simulink model "JT60_RCB_ACB-"  (R2015a)
settings: Solver=ode15s  StartTime=0.0  StopTime=1e3  MaxStep=1e2  RelTol=1e-3
libraries: simCryogenics_lib x146, nesl_utility x101
settings Model: Creator=GM246266  LastModifiedBy=FB229602
settings SimscapeCC: SimscapeLogType=all

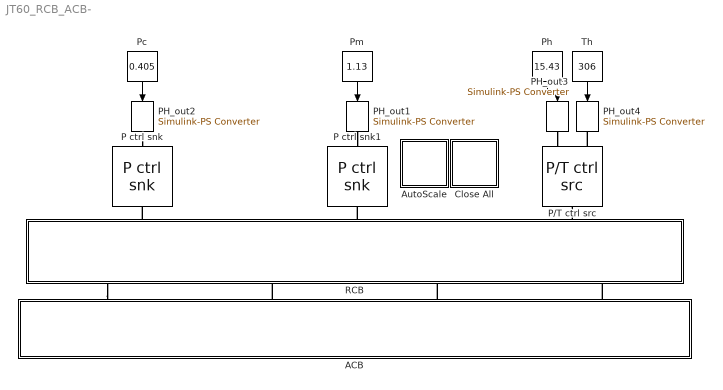
== system JT60_RCB_ACB- ==
  ACB : Subsystem
  AutoScale : Subsystem
      settings: OpenFcn=|
      | set(0, 'showhiddenhandles', 'on')
      | 
      | scope = findobj(0, 'Tag', 'SIMULINK_SIMSCOPE_FIGURE');
      | 
      | for i=1:length(scope)
      |   simscope('ScopeBar', 'ActionIcon', 'Find',     scope(i))
      | end
      | 
      | set(0, 'showhiddenhandles', 'off')
      mask Display: disp('Auto\nScale\nScope')
  Close All : Subsystem
      settings: OpenFcn=|
      | set(0, 'showhiddenhandles', 'on')
      | scope = findobj(0, 'Tag','SIMULINK_SIMSCOPE_FIGURE');
      | close(scope)
      | set(0, 'showhiddenhandles', 'off')
      mask Display: disp('Close\nAll\nScope')
  P ctrl snk : simCryogenics_lib/Sources_Sinks/P ctrl snk
  P ctrl snk1 : simCryogenics_lib/Sources_Sinks/P ctrl snk
  P/T ctrl src : simCryogenics_lib/Sources_Sinks/P//T ctrl src
  PH_out1 : nesl_utility/Simulink-PS Converter  PhysicalDomain=network_engine_domain  SubClassName=ps_input  LeftPortType=input  RightPortType=output  PseudoPeriodic=off  Frequencies=[]  NoiseDistribution=none  NoiseParameters=[]  Unit=bar  AffineConversion=off  InputFiltering=off  SimscapeFilterOrder=1  InputFilterTimeConstant=0.001  UdotUserProvided=1
  PH_out2 : nesl_utility/Simulink-PS Converter  PhysicalDomain=network_engine_domain  SubClassName=ps_input  LeftPortType=input  RightPortType=output  PseudoPeriodic=off  Frequencies=[]  NoiseDistribution=none  NoiseParameters=[]  Unit=bar  AffineConversion=off  InputFiltering=off  SimscapeFilterOrder=1  InputFilterTimeConstant=0.001  UdotUserProvided=1
  PH_out3 : nesl_utility/Simulink-PS Converter  PhysicalDomain=network_engine_domain  SubClassName=ps_input  LeftPortType=input  RightPortType=output  PseudoPeriodic=off  Frequencies=[]  NoiseDistribution=none  NoiseParameters=[]  Unit=bar  AffineConversion=off  InputFiltering=off  SimscapeFilterOrder=1  InputFilterTimeConstant=0.001  UdotUserProvided=1
  PH_out4 : nesl_utility/Simulink-PS Converter  PhysicalDomain=network_engine_domain  SubClassName=ps_input  LeftPortType=input  RightPortType=output  PseudoPeriodic=off  Frequencies=[]  NoiseDistribution=none  NoiseParameters=[]  Unit=K  AffineConversion=off  InputFiltering=off  SimscapeFilterOrder=1  InputFilterTimeConstant=0.001  UdotUserProvided=1
  Pc : Constant  Value=0.405
  Ph : Constant  Value=15.43
  Pm : Constant  Value=1.13
  RCB : Subsystem
  Th : Constant  Value=306
  wires:
  Th/1 -> PH_out4/1
  Ph/1 -> PH_out3/1
  Pm/1 -> PH_out1/1
  Pc/1 -> PH_out2/1
  connections:
  PH_out2/RConn1 -- P ctrl snk/LConn1
  PH_out1/RConn1 -- P ctrl snk1/LConn1
  PH_out3/RConn1 -- P/T ctrl src/LConn1
  P/T ctrl src/LConn2 -- PH_out4/RConn1
  RCB/RConn2 -- P ctrl snk1/RConn1
  RCB/RConn3 -- P/T ctrl src/RConn1
  RCB/RConn1 -- P ctrl snk/RConn1
  RCB/LConn1 -- ACB/RConn1
  ACB/RConn2 -- RCB/LConn2
  ACB/RConn3 -- RCB/LConn3
  ACB/RConn4 -- RCB/LConn4

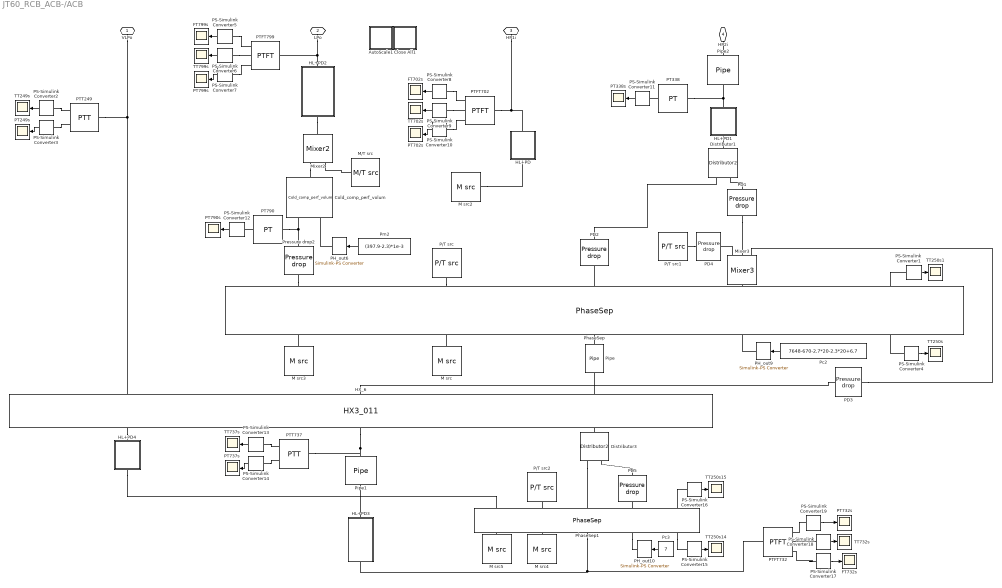
== system JT60_RCB_ACB-/ACB ==
  AutoScale1 : Subsystem
      settings: OpenFcn=|
      | set(0, 'showhiddenhandles', 'on')
      | 
      | scope = findobj(0, 'Tag', 'SIMULINK_SIMSCOPE_FIGURE');
      | 
      | for i=1:length(scope)
      |   simscope('ScopeBar', 'ActionIcon', 'Find',     scope(i))
      | end
      | 
      | set(0, 'showhiddenhandles', 'off')
      mask Display: disp('Auto\nScale\nScope')
  Close All1 : Subsystem
      settings: OpenFcn=|
      | set(0, 'showhiddenhandles', 'on')
      | scope = findobj(0, 'Tag','SIMULINK_SIMSCOPE_FIGURE');
      | close(scope)
      | set(0, 'showhiddenhandles', 'off')
      mask Display: disp('Close\nAll\nScope')
  Cold_comp_perf_volum : simCryogenics_lib/Elements/Cold_comp_perf_volum  P0=1.069 bar  eta=0.68  Sin_specify=off  Sin_priority=High  Sin=0 kJ/kg  HoutIs_specify=off  HoutIs_priority=High  HoutIs=0 kJ/kg
  Distributor1 : simCryogenics_lib/Elements/Distributor2
  Distributor3 : simCryogenics_lib/Elements/Distributor2
  FT702s : Scope
      settings: SaveName=FT
  FT732s : Scope
      settings: SaveName=FT732
  FT799s : Scope
      settings: SaveName=FT799
  HL+PD : Subsystem
  HL+PD1 : Subsystem
  HL+PD2 : Subsystem
  HL+PD3 : Subsystem
  HL+PD4 : Subsystem
  HX_6 : simCryogenics_lib/Elements/HX3_011  N=10  Vh=1 m^3  Vm=1 m^3  Vc=1 m^3  M=1000 kg  Kh=0.02/0.3068 s*bar/kg  Km=0.005/0.2835 s*bar/kg  Kc=0.02/0.02334 s*bar/kg  hh_m=865.4*(0.2835)/(0.2835+0.02334) J/s/K  hh_c=865.4*(0.02334)/(0.2835+0.02334) J/s/K  hm_c=1 J/s/K  Th0=4.4 K  Ph0=4.79 bar  Mh0=0.3068 kg/s  Tm0=3.7 K  Pm0=4.2 bar  Mm0=0.2835 kg/s  Tc0=3.661 K  Pc0=0.53 bar  Mc0=0.02334 kg/s  sensh=0  sensm=1  sensc=1
  M src{,3..5} (4 alike) : simCryogenics_lib/Sources_Sinks/M src  M=0 kg/s
  M src2 : simCryogenics_lib/Sources_Sinks/M src  M=0.020 kg/s
  M/T src : simCryogenics_lib/Sources_Sinks/M//T src  M=0.0023 kg/s  T=4.784 K
  Mixer2 : simCryogenics_lib/Elements/Mixer2
  Mixer3 : simCryogenics_lib/Elements/Mixer3
  P/T src : simCryogenics_lib/Sources_Sinks/P//T src  P=1 bar  T=300 K
  P/T src1 : simCryogenics_lib/Sources_Sinks/P//T src  P=4.44 bar  T=4.407 K
  P/T src2 : simCryogenics_lib/Sources_Sinks/P//T src  P=1 bar  T=300 K
  PD1 : simCryogenics_lib/Utilities/Pressure drop  K=3.771/0.09206 s*bar/kg
  PD2 : simCryogenics_lib/Utilities/Pressure drop  K=0.07/0.3068 s*bar/kg
  PD3 : simCryogenics_lib/Utilities/Pressure drop  K=3.106/0.2835 s*bar/kg
  PD4 : simCryogenics_lib/Utilities/Pressure drop  K=3.351/0.02 s*bar/kg
  PD5 : simCryogenics_lib/Utilities/Pressure drop  K=4.240/0.02334 s*bar/kg
  PH_out10 : nesl_utility/Simulink-PS Converter  PhysicalDomain=network_engine_domain  SubClassName=ps_input  LeftPortType=input  RightPortType=output  PseudoPeriodic=off  Frequencies=[]  NoiseDistribution=none  NoiseParameters=[]  Unit=1  AffineConversion=off  InputFiltering=off  SimscapeFilterOrder=1  InputFilterTimeConstant=0.001  UdotUserProvided=1
  PH_out6 : nesl_utility/Simulink-PS Converter  PhysicalDomain=network_engine_domain  SubClassName=ps_input  LeftPortType=input  RightPortType=output  PseudoPeriodic=off  Frequencies=[]  NoiseDistribution=none  NoiseParameters=[]  Unit=1  AffineConversion=off  InputFiltering=off  SimscapeFilterOrder=1  InputFilterTimeConstant=0.001  UdotUserProvided=1
  PH_out9 : nesl_utility/Simulink-PS Converter  PhysicalDomain=network_engine_domain  SubClassName=ps_input  LeftPortType=input  RightPortType=output  PseudoPeriodic=off  Frequencies=[]  NoiseDistribution=none  NoiseParameters=[]  Unit=1  AffineConversion=off  InputFiltering=off  SimscapeFilterOrder=1  InputFilterTimeConstant=0.001  UdotUserProvided=1
  PS-Simulink Converter{1..19} (19 alike) : nesl_utility/PS-Simulink Converter  PhysicalDomain=network_engine_domain  SubClassName=ps_output  LeftPortType=input  RightPortType=output  PseudoPeriodic=off  Frequencies=[]  Unit=1  AffineConversion=off
  PT249s : Scope
      settings: SaveName=PT
  PT338 : simCryogenics_lib/Sensors/PT
  PT338s : Scope
      settings: SaveName=PT1
  PT702s : Scope
      settings: SaveName=PT2
  PT732s : Scope
      settings: SaveName=PT732
  PT737s : Scope
      settings: SaveName=PT737
  PT790 : simCryogenics_lib/Sensors/PT
  PT790s : Scope
      settings: YMin=0  YMax=2.5  SaveName=PT790
  PT799s : Scope
      settings: SaveName=PT3
  PTFT702 : simCryogenics_lib/Sensors/PTFT
  PTFT732 : simCryogenics_lib/Sensors/PTFT
  PTFT799 : simCryogenics_lib/Sensors/PTFT
  PTT249 : simCryogenics_lib/Sensors/PTT
  PTT737 : simCryogenics_lib/Sensors/PTT
  Pc2 : Constant  Value=7648-670-2.7*20-2.3*20+6.7
  Pc3 : Constant  Value=7
  PhaseSep : simCryogenics_lib/Elements/PhaseSep  Ideal1=1  DeltaT1=1 K  N1=1  h1=1 W/K  Ideal2=1  DeltaT2=0.1 K  N2=1  h2=1 W/K  hmax=10 m  S=10 m^2  P0=1.089 bar  h0=50
  PhaseSep1 : simCryogenics_lib/Elements/PhaseSep  Ideal1=1  DeltaT1=1 K  N1=1  h1=1 W/K  Ideal2=1  DeltaT2=0.1 K  N2=1  h2=1 W/K  hmax=10 m  S=10 m^2  P0=0.53 bar  h0=50
  Pipe : simCryogenics_lib/Elements/Pipe  Vol=0.01 m^3  Ideal=1  P0=4.79 bar  T0=4.16 K
  Pipe1 : simCryogenics_lib/Elements/Pipe  Vol=0.01 m^3  Ideal=1  P0=4.195 bar  T0=4.16 K
  Pipe2 : simCryogenics_lib/Elements/Pipe  Vol=0.01 m^3  Ideal=1  P0=4.87 bar  T0=4.91 K
  Pm2 : Constant  Value=(397.9-2.3)*1e-3
  Pressure drop2 : simCryogenics_lib/Utilities/Pressure drop  K=0.02/((397.9-2.3)*1e-3) s*bar/kg
  TT249s : Scope
      settings: SaveName=TT249
  TT250s{,1,14..15} (4 alike) : Scope
      TT250s settings: TimeRange=100000  YMin=49.99  YMax=50.08000000000001  SaveName=TT
      TT250s1 settings: SaveName=TT1
      TT250s14 settings: TimeRange=24979.14205816138  YMin=48.2  YMax=49.7  SaveName=TT14
      TT250s15 settings: SaveName=TT15
  TT702s : Scope
      settings: SaveName=FT702
  TT732s : Scope
      settings: SaveName=TT732
  TT737s : Scope
      settings: SaveName=TT737
  TT799s : Scope
      settings: SaveName=TT799
  VLPo : PMIOPort  Port=1  Side=Right
  LPo : PMIOPort  Port=2  Side=Right
  HP1i : PMIOPort  Port=3  Side=Right
  HP2i : PMIOPort  Port=4  Side=Right
  wires:
  PS-Simulink Converter8/1 -> FT702s/1
  PS-Simulink Converter1/1 -> TT250s1/1
  Pc2/1 -> PH_out9/1
  PS-Simulink Converter4/1 -> TT250s/1
  PS-Simulink Converter15/1 -> TT250s14/1
  PS-Simulink Converter3/1 -> PT249s/1
  PS-Simulink Converter16/1 -> TT250s15/1
  PS-Simulink Converter6/1 -> TT799s/1
  PS-Simulink Converter2/1 -> TT249s/1
  Pc3/1 -> PH_out10/1
  PS-Simulink Converter5/1 -> FT799s/1
  PS-Simulink Converter9/1 -> TT702s/1
  PS-Simulink Converter13/1 -> TT737s/1
  PS-Simulink Converter12/1 -> PT790s/1
  PS-Simulink Converter11/1 -> PT338s/1
  PS-Simulink Converter7/1 -> PT799s/1
  PS-Simulink Converter18/1 -> TT732s/1
  PS-Simulink Converter14/1 -> PT737s/1
  PS-Simulink Converter19/1 -> PT732s/1
  PS-Simulink Converter10/1 -> PT702s/1
  PS-Simulink Converter17/1 -> FT732s/1
  Pm2/1 -> PH_out6/1
  connections:
  PT338/LConn1 -- HL+PD1/LConn1 -- Pipe2/RConn1
  HL+PD2/RConn1 -- LPo/RConn1 -- PTFT799/LConn1
  PTFT702/LConn1 -- HP1i/RConn1 -- HL+PD/LConn1
  PTT249/LConn1 -- HX_6/LConn1 -- VLPo/RConn1
  P/T src/RConn1 -- PhaseSep/LConn2
  HL+PD3/RConn1 -- Pipe1/LConn1
  HL+PD3/LConn1 -- PhaseSep1/RConn3 -- PTFT732/LConn1
  Mixer3/RConn1 -- PhaseSep/LConn4
  Cold_comp_perf_volum/LConn1 -- PT790/LConn1 -- Pressure drop2/RConn1
  HX_6/LConn3 -- Pipe/RConn1
  Distributor3/RConn2 -- PhaseSep1/LConn3
  PS-Simulink Converter8/LConn1 -- PTFT702/RConn3
  PS-Simulink Converter7/LConn1 -- PTFT799/RConn1
  HX_6/RConn3 -- Distributor3/LConn1
  PH_out6/RConn1 -- Cold_comp_perf_volum/LConn2
  PD5/RConn1 -- PhaseSep1/LConn4
  PS-Simulink Converter2/LConn1 -- PTT249/RConn2
  PS-Simulink Converter1/LConn1 -- PhaseSep/LConn5
  HL+PD4/LConn1 -- PhaseSep1/LConn1
  Mixer3/LConn3 -- PD4/RConn1
  M src3/RConn1 -- PhaseSep/RConn1
  HX_6/LConn2 -- PD3/LConn1
  PS-Simulink Converter16/LConn1 -- PhaseSep1/LConn5
  PD5/LConn1 -- Distributor3/RConn1
  PS-Simulink Converter5/LConn1 -- PTFT799/RConn3
  PS-Simulink Converter14/LConn1 -- PTT737/RConn1
  PS-Simulink Converter3/LConn1 -- PTT249/RConn1
  P/T src2/RConn1 -- PhaseSep1/LConn2
  PT790/RConn1 -- PS-Simulink Converter12/LConn1
  Pipe/LConn1 -- PhaseSep/RConn3
  PS-Simulink Converter4/LConn1 -- PhaseSep/RConn5
  PhaseSep/LConn3 -- PD2/RConn1
  PS-Simulink Converter6/LConn1 -- PTFT799/RConn2
  PD1/RConn1 -- Mixer3/LConn2
  HX_6/RConn1 -- HL+PD4/RConn1
  PS-Simulink Converter9/LConn1 -- PTFT702/RConn2
  PS-Simulink Converter18/LConn1 -- PTFT732/RConn2
  PH_out9/RConn1 -- PhaseSep/RConn4
  M src5/RConn1 -- PhaseSep1/RConn1
  PS-Simulink Converter10/LConn1 -- PTFT702/RConn1
  Pressure drop2/LConn1 -- PhaseSep/LConn1
  PS-Simulink Converter17/LConn1 -- PTFT732/RConn3
  M src2/RConn1 -- HL+PD/RConn1
  Distributor1/RConn2 -- PD2/LConn1
  P/T src1/RConn1 -- PD4/LConn1
  M src4/RConn1 -- PhaseSep1/RConn2
  PD3/RConn1 -- Mixer3/LConn1
  PS-Simulink Converter13/LConn1 -- PTT737/RConn2
  Distributor1/LConn1 -- HL+PD1/RConn1
  PT338/RConn1 -- PS-Simulink Converter11/LConn1
  PS-Simulink Converter19/LConn1 -- PTFT732/RConn1
  PhaseSep1/RConn4 -- PH_out10/RConn1
  Mixer2/LConn1 -- Cold_comp_perf_volum/RConn1
  PD1/LConn1 -- Distributor1/RConn1
  PhaseSep1/RConn5 -- PS-Simulink Converter15/LConn1
  Pipe1/RConn1 -- HX_6/RConn2 -- PTT737/LConn1
  M src/RConn1 -- PhaseSep/RConn2
  Pipe2/LConn1 -- HP2i/RConn1
  M/T src/RConn1 -- Mixer2/LConn2
  HL+PD2/LConn1 -- Mixer2/RConn1

== system JT60_RCB_ACB-/AutoScale ==

== system JT60_RCB_ACB-/Close All ==

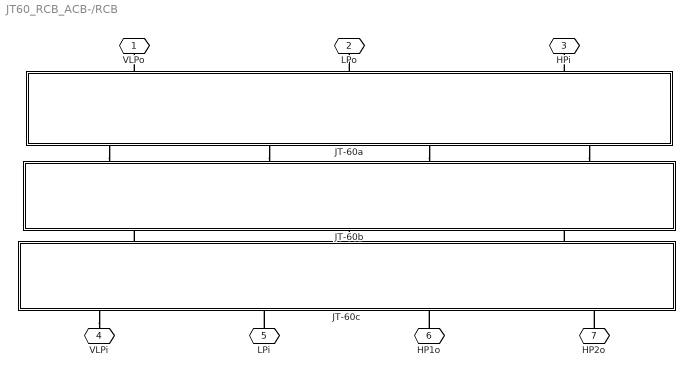
== system JT60_RCB_ACB-/RCB ==
  JT-60a : Subsystem
  JT-60b : Subsystem
  "JT-60c " : Subsystem
  VLPo : PMIOPort  Port=1  Side=Right
  LPo : PMIOPort  Port=2  Side=Right
  HPi : PMIOPort  Port=3  Side=Right
  VLPi : PMIOPort  Port=4  Side=Left
  LPi : PMIOPort  Port=5  Side=Left
  HP1o : PMIOPort  Port=6  Side=Left
  HP2o : PMIOPort  Port=7  Side=Left
  connections:
  JT-60a/LConn2 -- JT-60b/RConn2
  JT-60a/LConn3 -- JT-60b/RConn3
  JT-60a/LConn4 -- JT-60b/RConn4
  "JT-60c "/RConn2 -- JT-60b/LConn2
  "JT-60c "/RConn3 -- JT-60b/LConn3
  "JT-60c "/RConn1 -- JT-60b/LConn1
  HP2o/RConn1 -- "JT-60c "/LConn4
  "JT-60c "/LConn1 -- VLPi/RConn1
  LPi/RConn1 -- "JT-60c "/LConn2
  HP1o/RConn1 -- "JT-60c "/LConn3
  JT-60a/RConn1 -- VLPo/RConn1
  JT-60a/RConn2 -- LPo/RConn1
  JT-60a/RConn3 -- HPi/RConn1
  JT-60a/LConn1 -- JT-60b/RConn1

== system JT60_RCB_ACB-/ACB/AutoScale1 ==

== system JT60_RCB_ACB-/ACB/Close All1 ==

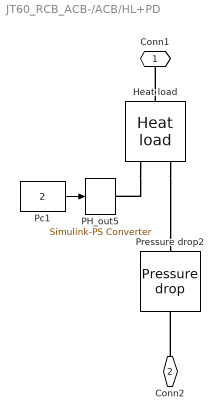
== system JT60_RCB_ACB-/ACB/HL+PD ==
  Heat load : simCryogenics_lib/Utilities/Heat load
  PH_out5 : nesl_utility/Simulink-PS Converter  PhysicalDomain=network_engine_domain  SubClassName=ps_input  LeftPortType=input  RightPortType=output  PseudoPeriodic=off  Frequencies=[]  NoiseDistribution=none  NoiseParameters=[]  Unit=J/s  AffineConversion=off  InputFiltering=off  SimscapeFilterOrder=1  InputFilterTimeConstant=0.001  UdotUserProvided=1
  Pc1 : Constant  Value=2
  Pressure drop2 : simCryogenics_lib/Utilities/Pressure drop  K=0.010/0.020 s*bar/kg
  Conn1 : PMIOPort  Port=1  Side=Right
  Conn2 : PMIOPort  Port=2  Side=Left
  wires:
  Pc1/1 -> PH_out5/1
  connections:
  Heat load/RConn1 -- Conn1/RConn1
  Conn2/RConn1 -- Pressure drop2/LConn1
  Heat load/LConn2 -- PH_out5/RConn1
  Heat load/LConn1 -- Pressure drop2/RConn1

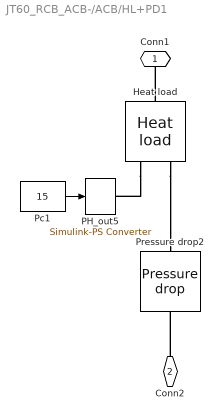
== system JT60_RCB_ACB-/ACB/HL+PD1 ==
  Heat load : simCryogenics_lib/Utilities/Heat load
  PH_out5 : nesl_utility/Simulink-PS Converter  PhysicalDomain=network_engine_domain  SubClassName=ps_input  LeftPortType=input  RightPortType=output  PseudoPeriodic=off  Frequencies=[]  NoiseDistribution=none  NoiseParameters=[]  Unit=J/s  AffineConversion=off  InputFiltering=off  SimscapeFilterOrder=1  InputFilterTimeConstant=0.001  UdotUserProvided=1
  Pc1 : Constant  Value=15
  Pressure drop2 : simCryogenics_lib/Utilities/Pressure drop  K=0.010/0.3989 s*bar/kg
  Conn1 : PMIOPort  Port=1  Side=Right
  Conn2 : PMIOPort  Port=2  Side=Left
  wires:
  Pc1/1 -> PH_out5/1
  connections:
  Heat load/RConn1 -- Conn1/RConn1
  Conn2/RConn1 -- Pressure drop2/LConn1
  Heat load/LConn2 -- PH_out5/RConn1
  Heat load/LConn1 -- Pressure drop2/RConn1

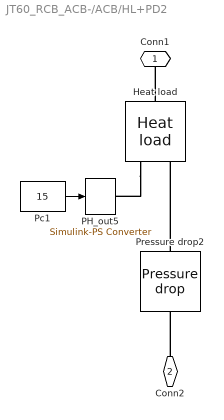
== system JT60_RCB_ACB-/ACB/HL+PD2 ==
  Heat load : simCryogenics_lib/Utilities/Heat load
  PH_out5 : nesl_utility/Simulink-PS Converter  PhysicalDomain=network_engine_domain  SubClassName=ps_input  LeftPortType=input  RightPortType=output  PseudoPeriodic=off  Frequencies=[]  NoiseDistribution=none  NoiseParameters=[]  Unit=J/s  AffineConversion=off  InputFiltering=off  SimscapeFilterOrder=1  InputFilterTimeConstant=0.001  UdotUserProvided=1
  Pc1 : Constant  Value=15
  Pressure drop2 : simCryogenics_lib/Utilities/Pressure drop  K=0.01/((397.9-2.3)*1e-3) s*bar/kg
  Conn1 : PMIOPort  Port=1  Side=Right
  Conn2 : PMIOPort  Port=2  Side=Left
  wires:
  Pc1/1 -> PH_out5/1
  connections:
  Heat load/RConn1 -- Conn1/RConn1
  Heat load/LConn2 -- PH_out5/RConn1
  Conn2/RConn1 -- Pressure drop2/LConn1
  Pressure drop2/RConn1 -- Heat load/LConn1

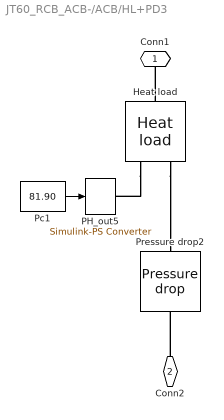
== system JT60_RCB_ACB-/ACB/HL+PD3 ==
  Heat load : simCryogenics_lib/Utilities/Heat load
  PH_out5 : nesl_utility/Simulink-PS Converter  PhysicalDomain=network_engine_domain  SubClassName=ps_input  LeftPortType=input  RightPortType=output  PseudoPeriodic=off  Frequencies=[]  NoiseDistribution=none  NoiseParameters=[]  Unit=J/s  AffineConversion=off  InputFiltering=off  SimscapeFilterOrder=1  InputFilterTimeConstant=0.001  UdotUserProvided=1
  Pc1 : Constant  Value=81.90
  Pressure drop2 : simCryogenics_lib/Utilities/Pressure drop  K=(0.5+0.07)/0.2835 s*bar/kg
  Conn1 : PMIOPort  Port=1  Side=Right
  Conn2 : PMIOPort  Port=2  Side=Left
  wires:
  Pc1/1 -> PH_out5/1
  connections:
  Heat load/LConn1 -- Pressure drop2/RConn1
  Heat load/LConn2 -- PH_out5/RConn1
  Conn2/RConn1 -- Pressure drop2/LConn1
  Heat load/RConn1 -- Conn1/RConn1

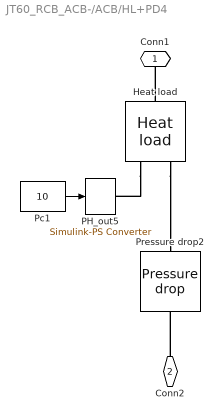
== system JT60_RCB_ACB-/ACB/HL+PD4 ==
  Heat load : simCryogenics_lib/Utilities/Heat load
  PH_out5 : nesl_utility/Simulink-PS Converter  PhysicalDomain=network_engine_domain  SubClassName=ps_input  LeftPortType=input  RightPortType=output  PseudoPeriodic=off  Frequencies=[]  NoiseDistribution=none  NoiseParameters=[]  Unit=J/s  AffineConversion=off  InputFiltering=off  SimscapeFilterOrder=1  InputFilterTimeConstant=0.001  UdotUserProvided=1
  Pc1 : Constant  Value=10
  Pressure drop2 : simCryogenics_lib/Utilities/Pressure drop  K=0.01/0.02334 s*bar/kg
  Conn1 : PMIOPort  Port=1  Side=Right
  Conn2 : PMIOPort  Port=2  Side=Left
  wires:
  Pc1/1 -> PH_out5/1
  connections:
  Heat load/LConn1 -- Pressure drop2/RConn1
  Heat load/LConn2 -- PH_out5/RConn1
  Conn2/RConn1 -- Pressure drop2/LConn1
  Heat load/RConn1 -- Conn1/RConn1

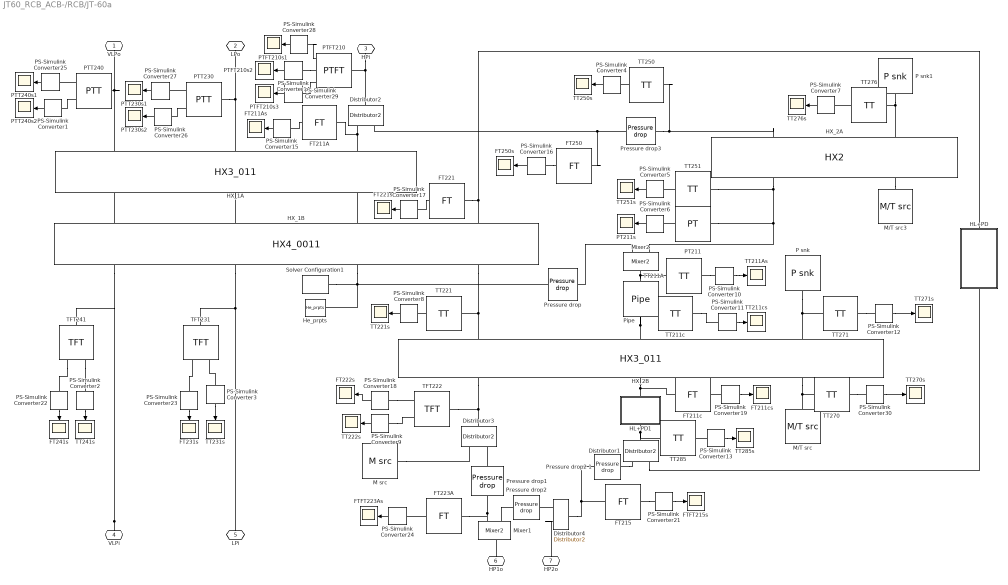
== system JT60_RCB_ACB-/RCB/JT-60a ==
  Distributor{1..4} (4 alike) : simCryogenics_lib/Elements/Distributor2
  FT211A : simCryogenics_lib/Sensors/FT
  FT211As : Scope
      settings: SaveName=FT211A
  FT211c : simCryogenics_lib/Sensors/FT
  FT211cs : Scope
      settings: SaveName=FT211c
  FT215 : simCryogenics_lib/Sensors/FT
  FT221 : simCryogenics_lib/Sensors/FT
  FT221s : Scope
      settings: SaveName=FT221
  FT222s : Scope
      settings: SaveName=FT222
  FT223A : simCryogenics_lib/Sensors/FT
  FT231s : Scope
      settings: SaveName=FT231
  FT241s : Scope
      settings: SaveName=FT241
  FT250 : simCryogenics_lib/Sensors/FT
  FT250s : Scope
      settings: SaveName=FT250
  FTFT215s : Scope
      settings: SaveName=FT215
  FTFT223As : Scope
      settings: SaveName=FT223A
  HL+PD : Subsystem
  HL+PD1 : Subsystem
  HX_1A : simCryogenics_lib/Elements/HX3_011  N=10  Vh=1 m^3  Vm=1 m^3  Vc=1 m^3  M=1000 kg  Kh=0 s*bar/kg  Km=0 s*bar/kg  Kc=0 s*bar/kg  hh_m=199100*0.585/(0.585+0.02334) J/s/K  hh_c=199100*0.02334/(0.585+0.02334) J/s/K  hm_c=1 J/s/K  Th0=306 K  Ph0=15.34 bar  Mh0=0.584 kg/s  Tm0=98 K  Pm0=1.130 bar  Mm0=0.589 kg/s  Tc0=98 K  Pc0=0.405 bar  Mc0=0.02334 kg/s  sensh=0  sensm=1  sensc=1
  HX_1B : simCryogenics_lib/Elements/HX4_0011  N=10  Vh=1 m^3  Vm=1 m^3  Vc=1 m^3  Vvc=1 m^3  M=1000 kg  Kh=0.03/0.425 s*bar/kg  Km=0.085/0.5925 s*bar/kg  Kc=0.135/0.589 s*bar/kg  Kvc=0.050/0.02334 s*bar/kg  hh_m=1 J/s/K  hh_c=17240*0.425/(0.425+0.584)*0.589/(0.589+0.02334) J/s/K  hh_vc=17240*0.425/(0.425+0.584)*0.02334/(0.589+0.02334) J/s/K  hm_c=17240*0.584/(0.425+0.584)*0.589/(0.589+0.02334) J/s/K  hm_vc=17240*0.584/(0.425+0.584)*0.02334/(0.589+0.02334) J/s/K  hc_vc=1 J/s/K  Th0=98 K  Ph0=15 bar  Mh0=0.425 kg/s  Tm0=99 K  Pm0=15 bar  Mm0=0.584 kg/s  Tc0=78 K  Pc0=1.1 bar  Mc0=0.589 kg/s  Tvc0=78 K  Pvc0=0.405 bar  Mvc0=0.02334 kg/s  sensh=0  sensm=0  sensc=1  sensvc=1
  HX_2A : simCryogenics_lib/Elements/HX2  N=10  Vh=1 m^3  Vc=1 m^3  M=1000 kg  Kh=0.05/0.04498 s*bar/kg  Kc=0 s*bar/kg  h=16470 J/s/K  Th0=300 K  Ph0=15 bar  Mc0=0.047*2 kg/s  Tc0=78 K  Pc0=1.1 bar  Mh0=0.047 kg/s
  HX_2B : simCryogenics_lib/Elements/HX3_011  N=10  Vh=1 m^3  Vm=1 m^3  Vc=1 m^3  M=1000 kg  Kh=0 s*bar/kg  Km=0.050/0.6374 s*bar/kg  Kc=0.030/0.425 s*bar/kg  hh_m=12710*0.6205/(0.6205+0.419) J/s/K  hh_c=12710*0.419/(0.6205+0.419) J/s/K  hm_c=1 J/s/K  Th0=78 K  Ph0=1.1 bar  Mh0=2 kg/s  Tm0=86.85 K  Pm0=15.33 bar  Mm0=0.6205 kg/s  Tc0=86.85 K  Pc0=15 bar  Mc0=0.419 kg/s  sensh=0  sensm=1  sensc=1
  He_prpts : simCryogenics_lib/Utilities/He_prpts  P_min=0.25 bar  T_min=3 K  T_max=320 K  P_max=20 bar  Mol=4.0026 * 10 ^ (- 3) kg/mol
  M src : simCryogenics_lib/Sources_Sinks/M src  M=6.6e-3 kg/s
  M/T src : simCryogenics_lib/Sources_Sinks/M//T src  M=4 kg/s  T=78 K
  M/T src3 : simCryogenics_lib/Sources_Sinks/M//T src  M=0.047*2 kg/s  T=78 K
  Mixer1 : simCryogenics_lib/Elements/Mixer2
  Mixer2 : simCryogenics_lib/Elements/Mixer2
  P snk : simCryogenics_lib/Sources_Sinks/P snk  P=1.1 bar
  P snk1 : simCryogenics_lib/Sources_Sinks/P snk  P=1.1 bar
  PS-Simulink Converter{1..19,21..30} (29 alike) : nesl_utility/PS-Simulink Converter  PhysicalDomain=network_engine_domain  SubClassName=ps_output  LeftPortType=input  RightPortType=output  PseudoPeriodic=off  Frequencies=[]  Unit=1  AffineConversion=off
  PT211 : simCryogenics_lib/Sensors/PT
  PT211s : Scope
      settings: SaveName=PT211
  PTFT210 : simCryogenics_lib/Sensors/PTFT
  PTFT210s1 : Scope
      settings: SaveName=FT210
  PTFT210s2 : Scope
      settings: SaveName=TT210
  PTFT210s3 : Scope
      settings: SaveName=PT210
  PTT230 : simCryogenics_lib/Sensors/PTT
  PTT230s1 : Scope
      settings: SaveName=TT230
  PTT230s2 : Scope
      settings: SaveName=PT230
  PTT240 : simCryogenics_lib/Sensors/PTT
  PTT240s1 : Scope
      settings: SaveName=TT240
  PTT240s2 : Scope
      settings: SaveName=PT240
  Pipe : simCryogenics_lib/Elements/Pipe  Vol=1 m^3  Ideal=0  P0=15.28 bar  T0=86.85 K
  Pressure drop : simCryogenics_lib/Utilities/Pressure drop  K=0.065/0.5925 s*bar/kg
  Pressure drop1 : simCryogenics_lib/Utilities/Pressure drop  K=0.010/0.4184 s*bar/kg
  "Pressure drop2 " : simCryogenics_lib/Utilities/Pressure drop  K=1.540/0.02108 s*bar/kg
  Pressure drop2 1 : simCryogenics_lib/Utilities/Pressure drop  K=0.04/0.2124 s*bar/kg
  Pressure drop3 : simCryogenics_lib/Utilities/Pressure drop  K=0.1/0.04498 s*bar/kg
  Solver Configuration1 : nesl_utility/Solver Configuration  PhysicalDomain=network_engine_domain  SubClassName=solver  LeftPortType=input  RightPortType=generic  Accelerate=off  Tones=[]  Harmonics=[]  SimulateNoise=off  Profile=off  UseLocalSampling=off  EnableSwitchedLinearOptims=on  FrequencyDomain=off  UseCCode=off  RelTol=0.001  AbsTol=1e-06  MinStep=1e-09  ToWorkspace=off  RevertToSquareIcSolve=off  NumHomotopyIterations=100  DoDC=off  ResidualTolerance=1e-09  UseLocalSolver=off  LocalSolverChoice=NE_BACKWARD_EULER_ADVANCER  LocalSolverSampleTime=5  DoFixedCost=off  MaxNonlinIter=10  MaxModeIter=2  LinearAlgebra=Sparse  DelaysMemoryBudget=1024  AutomaticFiltering=on  FilteringTimeConstant=0.001
  TFT222 : simCryogenics_lib/Sensors/TFT
  TFT231 : simCryogenics_lib/Sensors/TFT
  TFT241 : simCryogenics_lib/Sensors/TFT
  TT211A : simCryogenics_lib/Sensors/TT
  TT211As : Scope
      settings: SaveName=TT211A
  TT211c : simCryogenics_lib/Sensors/TT
  TT211cs : Scope
      settings: SaveName=TT211C
  TT{221,250..251,270..271,276,285} (7 alike) : simCryogenics_lib/Sensors/TT
  TT221s : Scope
      settings: SaveName=TT221
  TT222s : Scope
      settings: YMin=78.75  YMax=79.225  SaveName=TT222
  TT231s : Scope
      settings: SaveName=TT231
  TT241s : Scope
      settings: SaveName=TT241
  TT250s : Scope
      settings: SaveName=TT250
  TT251s : Scope
      settings: SaveName=TT251
  TT270s : Scope
      settings: SaveName=TT270
  TT271s : Scope
      settings: SaveName=TT271
  TT276s : Scope
      settings: SaveName=TT276
  TT285s : Scope
      settings: TimeRange=100000  SaveName=TT285
  VLPo : PMIOPort  Port=1  Side=Right
  LPo : PMIOPort  Port=2  Side=Right
  HPi : PMIOPort  Port=3  Side=Right
  VLPi : PMIOPort  Port=4  Side=Left
  LPi : PMIOPort  Port=5  Side=Left
  HP1o : PMIOPort  Port=6  Side=Left
  HP2o : PMIOPort  Port=7  Side=Left
  wires:
  PS-Simulink Converter2/1 -> TT241s/1
  PS-Simulink Converter3/1 -> TT231s/1
  PS-Simulink Converter4/1 -> TT250s/1
  PS-Simulink Converter5/1 -> TT251s/1
  PS-Simulink Converter6/1 -> PT211s/1
  PS-Simulink Converter7/1 -> TT276s/1
  PS-Simulink Converter8/1 -> TT221s/1
  PS-Simulink Converter9/1 -> TT222s/1
  PS-Simulink Converter10/1 -> TT211As/1
  PS-Simulink Converter11/1 -> TT211cs/1
  PS-Simulink Converter12/1 -> TT271s/1
  PS-Simulink Converter13/1 -> TT285s/1
  PS-Simulink Converter16/1 -> FT250s/1
  PS-Simulink Converter15/1 -> FT211As/1
  PS-Simulink Converter17/1 -> FT221s/1
  PS-Simulink Converter18/1 -> FT222s/1
  PS-Simulink Converter19/1 -> FT211cs/1
  PS-Simulink Converter22/1 -> FT241s/1
  PS-Simulink Converter23/1 -> FT231s/1
  PS-Simulink Converter21/1 -> FTFT215s/1
  PS-Simulink Converter24/1 -> FTFT223As/1
  PS-Simulink Converter25/1 -> PTT240s1/1
  PS-Simulink Converter1/1 -> PTT240s2/1
  PS-Simulink Converter27/1 -> PTT230s1/1
  PS-Simulink Converter26/1 -> PTT230s2/1
  PS-Simulink Converter28/1 -> PTFT210s1/1
  PS-Simulink Converter14/1 -> PTFT210s2/1
  PS-Simulink Converter29/1 -> PTFT210s3/1
  PS-Simulink Converter30/1 -> TT270s/1
  connections:
  HX_2A/RConn1 -- M/T src3/RConn1
  Mixer2/LConn2 -- PT211/LConn1 -- HX_2A/RConn2 -- TT251/LConn1
  HX_1B/LConn3 -- HX_1A/RConn3
  Distributor2/LConn1 -- HPi/RConn1 -- PTFT210/LConn1
  TT276/LConn1 -- P snk1/RConn1 -- HX_2A/LConn1
  HX_1B/LConn1 -- HX_1A/RConn1
  TT270/LConn1 -- HX_2B/LConn3 -- M/T src/RConn1
  Solver Configuration1/RConn1 -- HX_1B/RConn3 -- He_prpts/RConn1 -- Pressure drop/LConn1
  HX_1B/LConn2 -- HX_1A/RConn2
  HX_2B/RConn1 -- HX_1B/RConn4 -- TT221/LConn1
  HX_2B/RConn3 -- P snk/RConn1 -- TT271/LConn1
  Pressure drop/RConn1 -- Mixer2/LConn1
  Mixer2/RConn1 -- Pipe/LConn1 -- TT211A/LConn1
  Pressure drop3/LConn1 -- FT250/LConn1 -- Distributor2/RConn2
  HL+PD1/LConn1 -- HX_2B/LConn2 -- FT211c/LConn1
  FT221/LConn1 -- HX_1B/LConn4 -- HL+PD/RConn1
  TFT231/LConn1 -- HX_1B/RConn2 -- LPi/RConn1
  VLPi/RConn1 -- HX_1B/RConn1 -- TFT241/LConn1
  FT211A/LConn1 -- HX_1A/LConn3 -- Distributor2/RConn1
  PTT240/LConn1 -- HX_1A/LConn1 -- VLPo/RConn1
  PTT230/LConn1 -- HX_1A/LConn2 -- LPo/RConn1
  Distributor3/LConn1 -- HX_2B/LConn1 -- TFT222/LConn1
  Pressure drop3/RConn1 -- HX_2A/LConn2 -- TT250/LConn1
  Distributor1/RConn2 -- HL+PD/LConn1
  HL+PD1/RConn1 -- Distributor1/LConn1 -- TT285/LConn1
  M src/RConn1 -- Distributor3/RConn1
  Pressure drop1/LConn1 -- Distributor3/RConn2
  Distributor4/LConn1 -- FT215/LConn1 -- Pressure drop2 1/RConn1
  Distributor4/RConn1 -- "Pressure drop2 "/LConn1
  Distributor4/RConn2 -- HP2o/RConn1
  Mixer1/LConn1 -- Pressure drop1/RConn1 -- FT223A/LConn1
  "Pressure drop2 "/RConn1 -- Mixer1/LConn2
  HP1o/RConn1 -- Mixer1/RConn1
  Pressure drop2 1/LConn1 -- Distributor1/RConn1
  TFT241/RConn1 -- PS-Simulink Converter2/LConn1
  PS-Simulink Converter3/LConn1 -- TFT231/RConn1
  PS-Simulink Converter4/LConn1 -- TT250/RConn1
  TT251/RConn1 -- PS-Simulink Converter5/LConn1
  PT211/RConn1 -- PS-Simulink Converter6/LConn1
  TT276/RConn1 -- PS-Simulink Converter7/LConn1
  PS-Simulink Converter8/LConn1 -- TT221/RConn1
  PS-Simulink Converter9/LConn1 -- TFT222/RConn1
  TT211A/RConn1 -- PS-Simulink Converter10/LConn1
  TT211c/RConn1 -- PS-Simulink Converter11/LConn1
  TT211c/LConn1 -- HX_2B/RConn2 -- Pipe/RConn1
  TT271/RConn1 -- PS-Simulink Converter12/LConn1
  PS-Simulink Converter13/LConn1 -- TT285/RConn1
  PS-Simulink Converter16/LConn1 -- FT250/RConn1
  PS-Simulink Converter15/LConn1 -- FT211A/RConn1
  PS-Simulink Converter17/LConn1 -- FT221/RConn1
  PS-Simulink Converter19/LConn1 -- FT211c/RConn1
  TFT241/RConn2 -- PS-Simulink Converter22/LConn1
  PS-Simulink Converter23/LConn1 -- TFT231/RConn2
  FT215/RConn1 -- PS-Simulink Converter21/LConn1
  FT223A/RConn1 -- PS-Simulink Converter24/LConn1
  PTT240/RConn1 -- PS-Simulink Converter1/LConn1
  PTT240/RConn2 -- PS-Simulink Converter25/LConn1
  PTT230/RConn1 -- PS-Simulink Converter26/LConn1
  PTT230/RConn2 -- PS-Simulink Converter27/LConn1
  PS-Simulink Converter29/LConn1 -- PTFT210/RConn1
  PS-Simulink Converter14/LConn1 -- PTFT210/RConn2
  PS-Simulink Converter28/LConn1 -- PTFT210/RConn3
  TT270/RConn1 -- PS-Simulink Converter30/LConn1
  PS-Simulink Converter18/LConn1 -- TFT222/RConn2

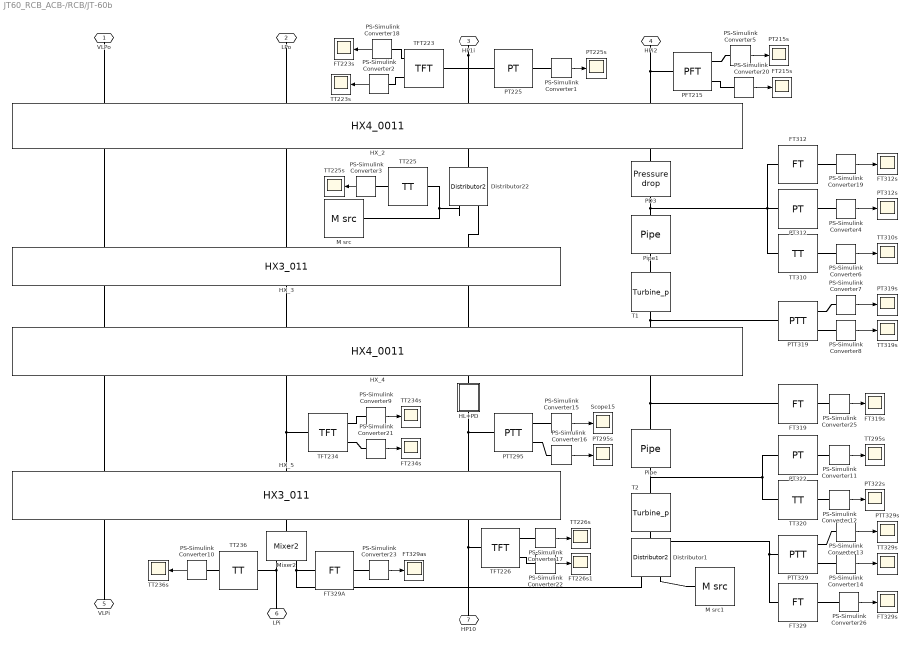
== system JT60_RCB_ACB-/RCB/JT-60b ==
  Distributor1 : simCryogenics_lib/Elements/Distributor2
  Distributor22 : simCryogenics_lib/Elements/Distributor2
  FT215s : Scope
      settings: SaveName=FT215B
  FT223s : Scope
      settings: SaveName=FT223
  FT226s1 : Scope
      settings: SaveName=FT226
  FT234s : Scope
      settings: SaveName=FT234
  FT312 : simCryogenics_lib/Sensors/FT
  FT312s : Scope
      settings: SaveName=FT312
  FT319 : simCryogenics_lib/Sensors/FT
  FT319s : Scope
      settings: SaveName=FT319
  FT329 : simCryogenics_lib/Sensors/FT
  FT329A : simCryogenics_lib/Sensors/FT
  FT329as : Scope
      settings: SaveName=FT329A
  FT329s : Scope
      settings: SaveName=FT329
  HL+PD : Subsystem
  HX_2 : simCryogenics_lib/Elements/HX4_0011  N=10  Vh=1 m^3  Vm=1 m^3  Vc=1 m^3  Vvc=1 m^3  M=1000 kg  Kh=0.020/0.1914 s*bar/kg  Km=0.020/(0.4184+0.02108) s*bar/kg  Kc=0.015/0.589 s*bar/kg  Kvc=0.0100/0.02334 s*bar/kg  hh_m=1 J/s/K  hh_c=73090*191/634*589/612 J/s/K  hh_vc=73090*191/634*23/612 J/s/K  hm_c=73090*443/634*589/612 J/s/K  hm_vc=73090*443/634*23/612 J/s/K  hc_vc=1 J/s/K  Th0=79 K  Ph0=15.43 bar  Mh0=0.1914 kg/s  Tm0=79 K  Pm0=15.43 bar  Mm0=0.4184+0.02108 kg/s  Tc0=38 K  Pc0=1.13 bar  Mc0=0.589 kg/s  Tvc0=38 K  Pvc0=0.405 bar  Mvc0=0.02334 kg/s  sensh=0  sensm=0  sensc=1  sensvc=1
  HX_3 : simCryogenics_lib/Elements/HX3_011  N=10  Vh=1 m^3  Vm=1 m^3  Vc=1 m^3  M=1000 kg  Kh=0.020/0.4198 s*bar/kg  Km=0.010/0.589 s*bar/kg  Kc=0.0050/0.02334 s*bar/kg  hh_m=17340*0.589/(0.589+0.02334) J/s/K  hh_c=17340*0.02334/(0.589+0.02334) J/s/K  hm_c=1 J/s/K  Th0=40 K  Ph0=13.5 bar  Mh0=0.4198 kg/s  Tm0=32 K  Pm0=1.29 bar  Mm0=0.589 kg/s  Tc0=32 K  Pc0=0.5 bar  Mc0=0.02334 kg/s  sensh=0  sensm=1  sensc=1
  HX_4 : simCryogenics_lib/Elements/HX4_0011  N=10  Vh=1 m^3  Vm=1 m^3  Vc=1 m^3  Vvc=1 m^3  M=1000 kg  Kh=0.050/0.1911 s*bar/kg  Km=0.020/0.4198 s*bar/kg  Kc=0.010/0.589 s*bar/kg  Kvc=0.005/0.02334 s*bar/kg  hh_m=1 J/s/K  hh_c=79510*191/611*589/612 J/s/K  hh_vc=7900*191/611*23/612 J/s/K  hm_c=79510*420/611*589/612 J/s/K  hm_vc=7900*420/611*23/612 J/s/K  hc_vc=1 J/s/K  Th0=31 K  Ph0=6.3 bar  Mh0=0.1911 kg/s  Tm0=31.22 K  Pm0=13.39 bar  Mm0=0.4198 kg/s  Tc0=18 K  Pc0=1.29 bar  Mc0=0.589 kg/s  Tvc0=18 K  Pvc0=0.47 bar  Mvc0=0.02334 kg/s  sensh=0  sensm=0  sensc=1  sensvc=1
  HX_5 : simCryogenics_lib/Elements/HX3_011  N=10  Vh=1 m^3  Vm=1 m^3  Vc=1 m^3  M=1000 kg  Kh=0.030/0.4198 s*bar/kg  Km=0.030/0.589 s*bar/kg  Kc=0.0150/0.02334 s*bar/kg  hh_m=51830*0.589/(0.589+0.2334) J/s/K  hh_c=51830*0.02334/(0.589+0.2334) J/s/K  hm_c=1 J/s/K  Th0=19 K  Ph0=13.3 bar  Mh0=0.4198 kg/s  Tm0=11 K  Pm0=1.3 bar  Mm0=0.589 kg/s  Tc0=11 K  Pc0=0.419 bar  Mc0=0.02334 kg/s  sensh=0  sensm=1  sensc=1
  M src : simCryogenics_lib/Sources_Sinks/M src  M=0.0197 kg/s
  M src1 : simCryogenics_lib/Sources_Sinks/M src  M=0.0003 kg/s
  Mixer2 : simCryogenics_lib/Elements/Mixer2
  PD3 : simCryogenics_lib/Utilities/Pressure drop  K=0.180/0.1914 s*bar/kg
  PFT215 : simCryogenics_lib/Sensors/PFT
  PS-Simulink Converter{1..23,25..26} (25 alike) : nesl_utility/PS-Simulink Converter  PhysicalDomain=network_engine_domain  SubClassName=ps_output  LeftPortType=input  RightPortType=output  PseudoPeriodic=off  Frequencies=[]  Unit=1  AffineConversion=off
  PT215s : Scope
      settings: SaveName=PT215
  PT225 : simCryogenics_lib/Sensors/PT
  PT225s : Scope
      settings: SaveName=PT225
  PT295s : Scope
      settings: SaveName=TT295
  PT312 : simCryogenics_lib/Sensors/PT
  PT312s : Scope
      settings: SaveName=PT312
  PT319s : Scope
      settings: SaveName=PT319
  PT322 : simCryogenics_lib/Sensors/PT
  PT322s : Scope
      settings: SaveName=TT320
  PTT295 : simCryogenics_lib/Sensors/PTT
  PTT319 : simCryogenics_lib/Sensors/PTT
  PTT329 : simCryogenics_lib/Sensors/PTT
  PTT329s : Scope
      settings: SaveName=PT329
  Pipe : simCryogenics_lib/Elements/Pipe  Vol=0.001 m^3  Ideal=0  P0=6.35 bar  T0=18 K
  Pipe1 : simCryogenics_lib/Elements/Pipe  Vol=1 m^3  Ideal=0  P0=14.76 bar  T0=40 K
  Scope15 : Scope
      settings: SaveName=PT295
  T1 : simCryogenics_lib/Elements/Turbine_p  A=5.2054e-05 m^2  D=0.03 m  Mass=0.02 kg  cst_eff=1  eta0=0.78  Tin0=40.07 K  Pin0=14.77 bar  Pout0=6.356 bar  N0=2000 1/s  Q0=0 W  v0=0  I=0 kg*m^2  gamma_specify=off  gamma_priority=High  gamma=0  C_specify=off  C_priority=High  C=0  Z_specify=off  Z_priority=High  Z=0  Cp_specify=off  Cp_priority=High  Cp=0 kJ/kg/K  Sin_specify=off  Sin_priority=High  Sin=0 kJ/kg  T_specify=off  T_priority=High  T=0 K  HoutIs_specify=off  HoutIs_priority=High  HoutIs=0 kJ/kg  u1_specify=off  u1_priority=High  u1=0 m/s  c1_specify=off  c1_priority=High  c1=0 m/s  v_specify=off  v_priority=High  v=0  eta_specify=off  eta_priority=High  eta=0  N_specify=off  N_priority=High  N=0 rad/s  Q_specify=off  Q_priority=High  Q=0 W
  T2 : simCryogenics_lib/Elements/Turbine_p  A=7.8987e-05 m^2  D=0.025 m  Mass=0.02 kg  cst_eff=1  eta0=0.76  Tin0=18.21 K  Pin0=6.307 bar  Pout0=1.350 bar  N0=2000 1/s  Q0=0 W  v0=0  I=0 kg*m^2  gamma_specify=off  gamma_priority=High  gamma=0  C_specify=off  C_priority=High  C=0  Z_specify=off  Z_priority=High  Z=0  Cp_specify=off  Cp_priority=High  Cp=0 kJ/kg/K  Sin_specify=off  Sin_priority=High  Sin=0 kJ/kg  T_specify=off  T_priority=High  T=0 K  HoutIs_specify=off  HoutIs_priority=High  HoutIs=0 kJ/kg  u1_specify=off  u1_priority=High  u1=0 m/s  c1_specify=off  c1_priority=High  c1=0 m/s  v_specify=off  v_priority=High  v=0  eta_specify=off  eta_priority=High  eta=0  N_specify=off  N_priority=High  N=0 rad/s  Q_specify=off  Q_priority=High  Q=0 W
  TFT223 : simCryogenics_lib/Sensors/TFT
  TFT226 : simCryogenics_lib/Sensors/TFT
  TFT234 : simCryogenics_lib/Sensors/TFT
  TT223s : Scope
      settings: SaveName=TT223
  TT{225,236,310,320} (4 alike) : simCryogenics_lib/Sensors/TT
  TT225s : Scope
      settings: SaveName=TT225
  TT226s : Scope
      settings: SaveName=TT226
  TT234s : Scope
      settings: SaveName=TT234
  TT236s : Scope
      settings: SaveName=TT236
  TT295s : Scope
      settings: YMin=6.35  YMax=6.54  SaveName=PT322
  TT310s : Scope
      settings: TimeRange=82572.12551127763  YMin=29.3  YMax=30.2  SaveName=TT310
  TT319s : Scope
      settings: YMin=30.2  YMax=31.6  SaveName=TT319
  TT329s : Scope
      settings: SaveName=TT329
  VLPo : PMIOPort  Port=1  Side=Right
  LPo : PMIOPort  Port=2  Side=Right
  HP1i : PMIOPort  Port=3  Side=Right
  HPi2 : PMIOPort  Port=4  Side=Right
  VLPi : PMIOPort  Port=5  Side=Left
  LPi : PMIOPort  Port=6  Side=Left
  HP10 : PMIOPort  Port=7  Side=Left
  wires:
  PS-Simulink Converter5/1 -> PT215s/1
  PS-Simulink Converter1/1 -> PT225s/1
  PS-Simulink Converter3/1 -> TT225s/1
  PS-Simulink Converter4/1 -> PT312s/1
  PS-Simulink Converter6/1 -> TT310s/1
  PS-Simulink Converter7/1 -> PT319s/1
  PS-Simulink Converter8/1 -> TT319s/1
  PS-Simulink Converter9/1 -> TT234s/1
  PS-Simulink Converter11/1 -> TT295s/1
  PS-Simulink Converter12/1 -> PT322s/1
  PS-Simulink Converter14/1 -> TT329s/1
  PS-Simulink Converter16/1 -> PT295s/1
  PS-Simulink Converter15/1 -> Scope15/1
  PS-Simulink Converter13/1 -> PTT329s/1
  PS-Simulink Converter10/1 -> TT236s/1
  PS-Simulink Converter17/1 -> TT226s/1
  PS-Simulink Converter21/1 -> FT234s/1
  PS-Simulink Converter23/1 -> FT329as/1
  PS-Simulink Converter19/1 -> FT312s/1
  PS-Simulink Converter25/1 -> FT319s/1
  PS-Simulink Converter26/1 -> FT329s/1
  PS-Simulink Converter2/1 -> TT223s/1
  PS-Simulink Converter18/1 -> FT223s/1
  PS-Simulink Converter20/1 -> FT215s/1
  PS-Simulink Converter22/1 -> FT226s1/1
  connections:
  TFT234/LConn1 -- HX_4/RConn2 -- HX_5/LConn2
  HX_5/RConn2 -- Mixer2/RConn1
  HX_4/LConn1 -- HX_3/RConn1
  HX_4/LConn2 -- HX_3/RConn2
  HX_4/LConn3 -- HX_3/RConn3
  HX_4/RConn1 -- HX_5/LConn1
  HX_2/RConn2 -- HX_3/LConn2
  HX_2/RConn1 -- HX_3/LConn1
  Distributor1/RConn2 -- FT329A/LConn1 -- Mixer2/LConn2
  Pipe1/RConn1 -- T1/LConn1
  T1/RConn1 -- HX_4/LConn4 -- PTT319/LConn1
  Pipe/LConn1 -- HX_4/RConn4 -- FT319/LConn1
  PT322/LConn1 -- Pipe/RConn1 -- T2/LConn1 -- TT320/LConn1
  HX_2/LConn1 -- VLPo/RConn1
  HP1i/RConn1 -- HX_2/LConn3 -- PT225/LConn1 -- TFT223/LConn1
  PFT215/LConn1 -- HX_2/LConn4 -- HPi2/RConn1
  HX_2/LConn2 -- LPo/RConn1
  HX_5/RConn1 -- VLPi/RConn1
  TFT226/LConn1 -- HX_5/RConn3 -- HP10/RConn1
  LPi/RConn1 -- TT236/LConn1 -- Mixer2/LConn1
  HX_2/RConn3 -- Distributor22/LConn1
  Distributor22/RConn2 -- M src/RConn1 -- TT225/LConn1
  HX_3/LConn3 -- Distributor22/RConn1
  HX_4/RConn3 -- HL+PD/LConn1
  PTT295/LConn1 -- HX_5/LConn3 -- HL+PD/RConn1
  HX_2/RConn4 -- PD3/LConn1
  Distributor1/LConn1 -- FT329/LConn1 -- PTT329/LConn1 -- T2/RConn1
  M src1/RConn1 -- Distributor1/RConn1
  PFT215/RConn1 -- PS-Simulink Converter5/LConn1
  PS-Simulink Converter1/LConn1 -- PT225/RConn1
  TFT223/RConn1 -- PS-Simulink Converter2/LConn1
  TT225/RConn1 -- PS-Simulink Converter3/LConn1
  PT312/RConn1 -- PS-Simulink Converter4/LConn1
  PS-Simulink Converter6/LConn1 -- TT310/RConn1
  PTT319/RConn1 -- PS-Simulink Converter7/LConn1
  PTT319/RConn2 -- PS-Simulink Converter8/LConn1
  PS-Simulink Converter9/LConn1 -- TFT234/RConn1
  PS-Simulink Converter12/LConn1 -- TT320/RConn1
  PT322/RConn1 -- PS-Simulink Converter11/LConn1
  PTT329/RConn1 -- PS-Simulink Converter13/LConn1
  PTT329/RConn2 -- PS-Simulink Converter14/LConn1
  PTT295/RConn2 -- PS-Simulink Converter16/LConn1
  PS-Simulink Converter15/LConn1 -- PTT295/RConn1
  TT236/RConn1 -- PS-Simulink Converter10/LConn1
  TFT226/RConn1 -- PS-Simulink Converter17/LConn1
  PT312/LConn1 -- TT310/LConn1 -- FT312/LConn1 -- PD3/RConn1 -- Pipe1/LConn1
  TFT234/RConn2 -- PS-Simulink Converter21/LConn1
  PS-Simulink Converter23/LConn1 -- FT329A/RConn1
  PS-Simulink Converter19/LConn1 -- FT312/RConn1
  PS-Simulink Converter25/LConn1 -- FT319/RConn1
  PS-Simulink Converter26/LConn1 -- FT329/RConn1
  PS-Simulink Converter18/LConn1 -- TFT223/RConn2
  PS-Simulink Converter20/LConn1 -- PFT215/RConn2
  PS-Simulink Converter22/LConn1 -- TFT226/RConn2

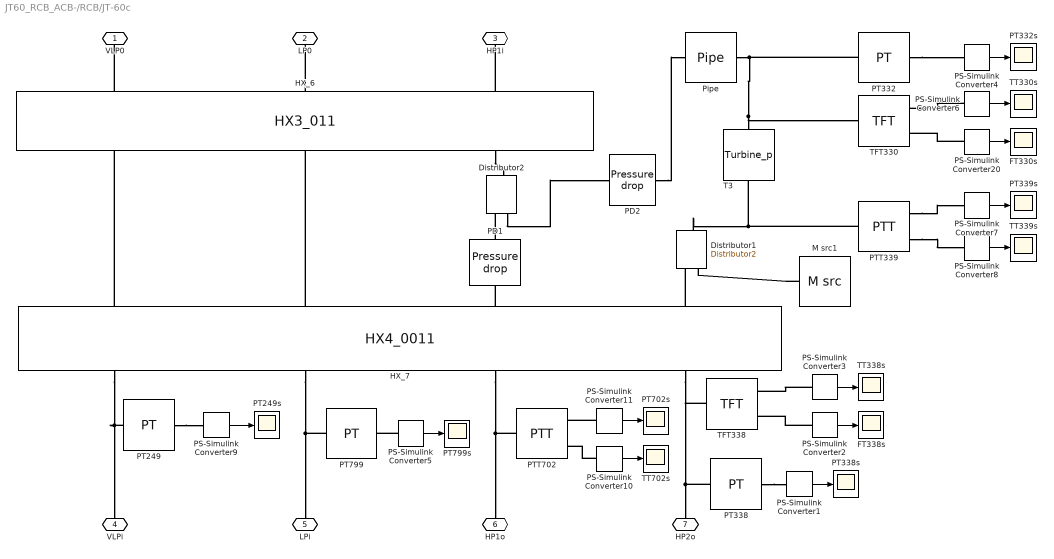
== system JT60_RCB_ACB-/RCB/JT-60c  ==
  Distributor1 : simCryogenics_lib/Elements/Distributor2
  Distributor2 : simCryogenics_lib/Elements/Distributor2
  FT330s : Scope
      settings: SaveName=FT330
  FT338s : Scope
      settings: SaveName=FT338
  HX_6 : simCryogenics_lib/Elements/HX3_011  N=10  Vh=1 m^3  Vm=1 m^3  Vc=1 m^3  M=1000 kg  Kh=0.010/0.4198 s*bar/kg  Km=0.005/(0.589-0.1911) s*bar/kg  Kc=0.005/0.02334 s*bar/kg  hh_m=22750*(0.598-0.1911)/(0.598-0.1911+0.02334) J/s/K  hh_c=22750*(0.02334)/(0.598-0.1911+0.02334) J/s/K  hm_c=1 J/s/K  Th0=11.64 K  Ph0=13.16 bar  Mh0=0.4198 kg/s  Tm0=6 K  Pm0=1.34 bar  Mm0=0.598-0.1911 kg/s  Tc0=6 K  Pc0=0.495 bar  Mc0=0.02334 kg/s  sensh=0  sensm=1  sensc=1
  HX_7 : simCryogenics_lib/Elements/HX4_0011  N=10  Vh=1 m^3  Vm=1 m^3  Vc=1 m^3  Vvc=1 m^3  M=1000 kg  Kh=0.010/0.3998 s*bar/kg  Km=0.005/0.020 s*bar/kg  Kc=0.005/0.3979 s*bar/kg  Kvc=0.005/0.2334 s*bar/kg  hh_m=1 J/s/K  hh_c=13770*0.3998/(0.3998+0.02)*0.3979/(0.3979+0.02334) J/s/K  hh_vc=13770*0.3998/(0.3998+0.02)*0.02334/(0.3979+0.02334) J/s/K  hm_c=13770*0.02/(0.3998+0.02)*0.3979/(0.3979+0.02334) J/s/K  hm_vc=13770*0.02/(0.3998+0.02)*0.02334/(0.3979+0.02334) J/s/K  hc_vc=1 J/s/K  Th0=6 K  Ph0=4 bar  Mh0=0.3998 kg/s  Tm0=7.7 K  Pm0=13.39 bar  Mm0=0.02 kg/s  Tc0=4.78 K  Pc0=1.29 bar  Mc0=0.3979 kg/s  Tvc0=4.5 K  Pvc0=0.5 bar  Mvc0=0.02334 kg/s  sensh=0  sensm=0  sensc=1  sensvc=1
  M src1 : simCryogenics_lib/Sources_Sinks/M src  M=0.00073 kg/s
  PD1 : simCryogenics_lib/Utilities/Pressure drop  K=5/0.020 s*bar/kg
  PD2 : simCryogenics_lib/Utilities/Pressure drop  K=0.080/0.3998 s*bar/kg
  PS-Simulink Converter{1..11,20} (12 alike) : nesl_utility/PS-Simulink Converter  PhysicalDomain=network_engine_domain  SubClassName=ps_output  LeftPortType=input  RightPortType=output  PseudoPeriodic=off  Frequencies=[]  Unit=1  AffineConversion=off
  PT{249,332,338,799} (4 alike) : simCryogenics_lib/Sensors/PT
  PT249s : Scope
      settings: SaveName=PT249
  PT332s : Scope
      settings: SaveName=PT332
  PT338s : Scope
      settings: YMin=-1.66533e-16  YMax=2.4  SaveName=PT338
  PT339s : Scope
      settings: SaveName=PT339
  PT702s : Scope
      settings: SaveName=PT702
  PT799s : Scope
      settings: SaveName=PT799
  PTT339 : simCryogenics_lib/Sensors/PTT
  PTT702 : simCryogenics_lib/Sensors/PTT
  Pipe : simCryogenics_lib/Elements/Pipe  Vol=1 m^3  Ideal=0  P0=13.05 bar  T0=7.2 K
  T3 : simCryogenics_lib/Elements/Turbine_p  A=4.0044e-05 m^2  D=0.01 m  Mass=0.02 kg  cst_eff=1  eta0=0.72  Tin0=7.295 K  Pin0=13.07 bar  Pout0=4.880 bar  N0=2000 1/s  Q0=0 W  v0=0  I=0 kg*m^2  gamma_specify=off  gamma_priority=High  gamma=0  C_specify=off  C_priority=High  C=0  Z_specify=off  Z_priority=High  Z=0  Cp_specify=off  Cp_priority=High  Cp=0 kJ/kg/K  Sin_specify=off  Sin_priority=High  Sin=0 kJ/kg  T_specify=off  T_priority=High  T=0 K  HoutIs_specify=off  HoutIs_priority=High  HoutIs=0 kJ/kg  u1_specify=off  u1_priority=High  u1=0 m/s  c1_specify=off  c1_priority=High  c1=0 m/s  v_specify=off  v_priority=High  v=0  eta_specify=off  eta_priority=High  eta=0  N_specify=off  N_priority=High  N=0 rad/s  Q_specify=off  Q_priority=High  Q=0 W
  TFT330 : simCryogenics_lib/Sensors/TFT
  TFT338 : simCryogenics_lib/Sensors/TFT
  TT330s : Scope
      settings: SaveName=TT330
  TT338s : Scope
      settings: SaveName=TT338
  TT339s : Scope
      settings: SaveName=TT339
  TT702s : Scope
      settings: SaveName=TT702
  VLP0 : PMIOPort  Port=1  Side=Right
  LP0 : PMIOPort  Port=2  Side=Right
  "HP1i " : PMIOPort  Port=3  Side=Right
  VLPi : PMIOPort  Port=4  Side=Left
  LPi : PMIOPort  Port=5  Side=Left
  HP1o : PMIOPort  Port=6  Side=Left
  HP2o : PMIOPort  Port=7  Side=Left
  wires:
  PS-Simulink Converter4/1 -> PT332s/1
  PS-Simulink Converter6/1 -> TT330s/1
  PS-Simulink Converter7/1 -> PT339s/1
  PS-Simulink Converter8/1 -> TT339s/1
  PS-Simulink Converter1/1 -> PT338s/1
  PS-Simulink Converter20/1 -> FT330s/1
  PS-Simulink Converter3/1 -> TT338s/1
  PS-Simulink Converter2/1 -> FT338s/1
  PS-Simulink Converter9/1 -> PT249s/1
  PS-Simulink Converter5/1 -> PT799s/1
  PS-Simulink Converter11/1 -> PT702s/1
  PS-Simulink Converter10/1 -> TT702s/1
  connections:
  HX_6/LConn3 -- "HP1i "/RConn1
  HX_7/RConn4 -- TFT338/LConn1 -- PT338/LConn1 -- HP2o/RConn1
  PT249/LConn1 -- HX_7/RConn1 -- VLPi/RConn1
  HX_6/LConn1 -- VLP0/RConn1
  HX_7/LConn1 -- HX_6/RConn1
  HX_6/LConn2 -- LP0/RConn1
  PT332/LConn1 -- TFT330/LConn1 -- T3/LConn1 -- Pipe/RConn1
  PTT702/LConn1 -- HX_7/RConn3 -- HP1o/RConn1
  PT799/LConn1 -- HX_7/RConn2 -- LPi/RConn1
  HX_7/LConn4 -- Distributor1/RConn2
  HX_6/RConn3 -- Distributor2/LConn1
  HX_7/LConn2 -- HX_6/RConn2
  HX_7/LConn3 -- PD1/RConn1
  Distributor2/RConn1 -- PD2/LConn1
  PD1/LConn1 -- Distributor2/RConn2
  Distributor1/LConn1 -- PTT339/LConn1 -- T3/RConn1
  M src1/RConn1 -- Distributor1/RConn1
  PTT339/RConn1 -- PS-Simulink Converter7/LConn1
  PS-Simulink Converter6/LConn1 -- TFT330/RConn1
  PT332/RConn1 -- PS-Simulink Converter4/LConn1
  PTT339/RConn2 -- PS-Simulink Converter8/LConn1
  PT338/RConn1 -- PS-Simulink Converter1/LConn1
  PD2/RConn1 -- Pipe/LConn1
  PS-Simulink Converter20/LConn1 -- TFT330/RConn2
  PS-Simulink Converter3/LConn1 -- TFT338/RConn1
  PS-Simulink Converter2/LConn1 -- TFT338/RConn2
  PT249/RConn1 -- PS-Simulink Converter9/LConn1
  PS-Simulink Converter5/LConn1 -- PT799/RConn1
  PS-Simulink Converter11/LConn1 -- PTT702/RConn1
  PS-Simulink Converter10/LConn1 -- PTT702/RConn2

== system JT60_RCB_ACB-/RCB/JT-60a/HL+PD ==
  Heat load : simCryogenics_lib/Utilities/Heat load
  PH_out5 : nesl_utility/Simulink-PS Converter  PhysicalDomain=network_engine_domain  SubClassName=ps_input  LeftPortType=input  RightPortType=output  PseudoPeriodic=off  Frequencies=[]  NoiseDistribution=none  NoiseParameters=[]  Unit=J/s  AffineConversion=off  InputFiltering=off  SimscapeFilterOrder=1  InputFilterTimeConstant=0.001  UdotUserProvided=1
  Pc1 : Constant  Value=4.410e4
  Pressure drop2 : simCryogenics_lib/Utilities/Pressure drop  K=(1.5+0.01)/0.425 s*bar/kg
  Conn1 : PMIOPort  Port=1  Side=Right
  Conn2 : PMIOPort  Port=2  Side=Left
  wires:
  Pc1/1 -> PH_out5/1
  connections:
  Heat load/RConn1 -- Conn1/RConn1
  Conn2/RConn1 -- Pressure drop2/LConn1
  Heat load/LConn2 -- PH_out5/RConn1
  Heat load/LConn1 -- Pressure drop2/RConn1

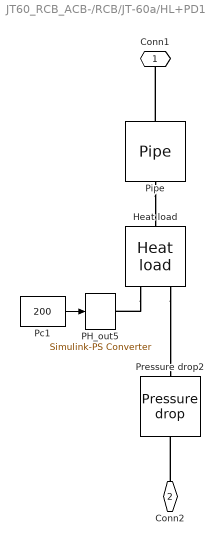
== system JT60_RCB_ACB-/RCB/JT-60a/HL+PD1 ==
  Heat load : simCryogenics_lib/Utilities/Heat load
  PH_out5 : nesl_utility/Simulink-PS Converter  PhysicalDomain=network_engine_domain  SubClassName=ps_input  LeftPortType=input  RightPortType=output  PseudoPeriodic=off  Frequencies=[]  NoiseDistribution=none  NoiseParameters=[]  Unit=J/s  AffineConversion=off  InputFiltering=off  SimscapeFilterOrder=1  InputFilterTimeConstant=0.001  UdotUserProvided=1
  Pc1 : Constant  Value=200
  Pipe : simCryogenics_lib/Elements/Pipe  Vol=1 m^3  Ideal=0  P0=15.23 bar  T0=80 K
  Pressure drop2 : simCryogenics_lib/Utilities/Pressure drop  K=0.220/0.6374 s*bar/kg
  Conn1 : PMIOPort  Port=1  Side=Right
  Conn2 : PMIOPort  Port=2  Side=Left
  wires:
  Pc1/1 -> PH_out5/1
  connections:
  Heat load/LConn1 -- Pressure drop2/RConn1
  Heat load/LConn2 -- PH_out5/RConn1
  Conn2/RConn1 -- Pressure drop2/LConn1
  Pipe/LConn1 -- Heat load/RConn1
  Pipe/RConn1 -- Conn1/RConn1

== system JT60_RCB_ACB-/RCB/JT-60b/HL+PD ==
  Heat load : simCryogenics_lib/Utilities/Heat load
  PH_out5 : nesl_utility/Simulink-PS Converter  PhysicalDomain=network_engine_domain  SubClassName=ps_input  LeftPortType=input  RightPortType=output  PseudoPeriodic=off  Frequencies=[]  NoiseDistribution=none  NoiseParameters=[]  Unit=J/s  AffineConversion=off  InputFiltering=off  SimscapeFilterOrder=1  InputFilterTimeConstant=0.001  UdotUserProvided=1
  Pc1 : Constant  Value=100
  Pressure drop2 : simCryogenics_lib/Utilities/Pressure drop  K=0.180/0.4198 s*bar/kg
  Conn1 : PMIOPort  Port=1  Side=Right
  Conn2 : PMIOPort  Port=2  Side=Left
  wires:
  Pc1/1 -> PH_out5/1
  connections:
  Heat load/RConn1 -- Conn1/RConn1
  Conn2/RConn1 -- Pressure drop2/LConn1
  Heat load/LConn2 -- PH_out5/RConn1
  Heat load/LConn1 -- Pressure drop2/RConn1
